simulink model "example1"  (R2015a)
settings: Solver=ode3  SolverMode=SingleTasking  StartTime=0.0  StopTime=10.0  RelTol=1e-3
libraries: simulink x2
settings Model: CovSFcnEnable=off  ExtModeTrigDuration=2  Creator=Cosmin  LastModifiedBy=kkhoo
settings OptimizationCC: OptimizeModelRefInitCode=on  LifeSpan=1
settings DebuggingCC: UnderspecifiedInitializationDetection=Classic  MergeDetectMultiDrivingBlocksExec=none
settings HardwareCC: ProdBitPerInt=16  ProdBitPerPointer=8  ProdIntDivRoundTo=Zero  ProdEndianess=LittleEndian  ProdWordSize=8  ProdHWDeviceType=Atmel->AVR
settings RTWCC: SystemTargetFile=realtime.tlc  GenerateMakefile=off  TemplateMakefile=realtime.tmf  Description=Run on Target Hardware  RTWVerbose=off  CustomSource=src/Engduino.h src/engduino_wrappers.cpp
settings ERTTargetCC: CombineOutputUpdateFcns=off  ExtModeTransport=3  ExtModeMexFile=ext_serial_win32_comm  ExtModeMexArgs=0 1 9600  ERTSrcFileBannerTemplate=realtime_code_template.cgt  ERTHdrFileBannerTemplate=realtime_code_template.cgt  ERTDataSrcFileTemplate=realtime_code_template.cgt  ERTDataHdrFileTemplate=realtime_code_template.cgt  ERTCustomFileTemplate=realtime_file_process.tlc

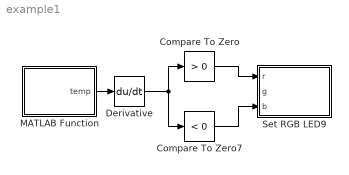
== system example1 ==
  Compare To Zero : simulink/Logic and Bit Operations/Compare To Zero  relop=>  OutDataTypeStr=uint8
  Compare To Zero7 : simulink/Logic and Bit Operations/Compare To Zero  relop=<  OutDataTypeStr=uint8
  Derivative : Derivative
  MATLAB Function : MATLAB Function  LoadFcn=|  TreatAsAtomicUnit=on  mask(Thermistor){}
      | set_param(gcs, 'CustomSource', strjoin(unique([strsplit(get_param(gcs, 'CustomSource')) ...
      |  'src/engduino_wrappers.cpp' 'src/Engduino.h'])));
      mask help: Outputs the temperature in milli degrees celsius.
  Set RGB LED9 : MATLAB Function  LoadFcn=|  TreatAsAtomicUnit=on  mask(RGB LED){led_index=1}
      | set_param(gcs, 'CustomSource', strjoin(unique([strsplit(get_param(gcs, 'CustomSource')) ...
      |  'src/engduino_wrappers.cpp' 'src/Engduino.h'])));
      mask prompts: led_index "LED index"
      mask help:
      | Control the Red, Green and Blue color values of the LED specified by the LED index parameter.
      | Both the LED index and the three color values are of type uint8 and must be in the range 0-15.
      settings: AttributesFormatString=LED %<led_index>
  wires:
  Derivative/1 -> Compare To Zero7/1, Compare To Zero/1
  MATLAB Function/1(temp) -> Derivative/1
  Compare To Zero/1 -> Set RGB LED9/1(r)
  Compare To Zero7/1 -> Set RGB LED9/3(b)

== matlab function example1/MATLAB Function ==
  data: temp output
function temp = thermistor()

temp = 0.0;

if strcmp(coder.target, 'rtw')
    temp = coder.ceval('thermistor_wrapper');
end

== matlab function example1/Set RGB LED9 ==
  data: led_index parameter uint8 [0..15]; r input uint8 [0..15]; g input uint8 [0..15]; b input uint8 [0..15]
function rgb_led(led_index, r, g, b)

if strcmp(coder.target, 'rtw')
    coder.ceval('rgb_leds_wrapper', led_index, r, g, b);
end
